simulink model "att2dcm"  (R2018a)
settings: Solver=VariableStepAuto  StartTime=0.0  StopTime=10.0  RelTol=1e-3
settings Model: Creator=lamy  LastModifiedBy=lamy

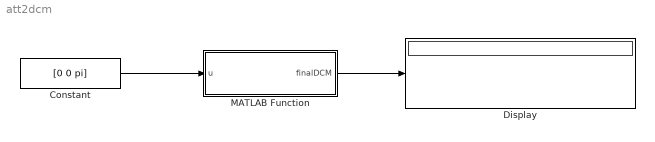
== system att2dcm ==
  Constant : Constant  Value=[0 0 pi]
  Display : Display
  MATLAB Function : MATLAB Function  TreatAsAtomicUnit=on
  wires:
  MATLAB Function/1(finalDCM) -> Display/1
  Constant/1 -> MATLAB Function/1(u)

== matlab function att2dcm/MATLAB Function ==
  data: u input; finalDCM output
function finalDCM = att2dcm(u)
yawDCM = [ cos(u(3)) sin(u(3)) 0 ;
-sin(u(3)) cos(u(3)) 0 ;
0 0 1 ];
pitchDCM = [ cos(u(2)) 0 -sin(u(2));
0 1 0 ;
sin(u(2)) 0 cos(u(2)) ];
rollDCM = [ 1 0 0 ;
0 cos(u(1)) sin(u(1));
0 -sin(u(1)) cos(u(1)) ];
finalDCM = rollDCM * pitchDCM * yawDCM;
